simulink model "LAB2_DigitalInput_Output"  (R2024a)
settings: Solver=FixedStepAuto  StartTime=0.0  StopTime=inf  FixedStep=1e-3  RelTol=1e-3  EnableMultiTasking=on
libraries: arduinolib x3
settings Model: ExtModeTrigDuration=2  Creator=VICTUS  LastModifiedBy=VICTUS
settings SolverCC: AutoInsertRateTranBlk=on
settings OptimizationCC: EnhancedBackFolding=on  PassReuseOutputArgsAs=Individual arguments  ZeroExternalMemoryAtStartup=off  ZeroInternalMemoryAtStartup=off  MaxStackSize=64  OptimizeBlockOrder=speed  DifferentSizesBufferReuse=on  OptimizationCustomize=off  EfficientTunableParamExpr=on
settings DebuggingCC: MultiTaskCondExecSysMsg=none  ParameterTunabilityLossMsg=error
settings HardwareCC: ProdBitPerPointer=32  ProdBitPerSizeT=32  ProdBitPerPtrDiffT=32  ProdLargestAtomicInteger=Long  ProdLargestAtomicFloat=Double  ProdWordSize=32  ProdHWDeviceType=ARM Compatible->ARM Cortex
settings SFSimCC: MATLABDynamicMemAlloc=off
settings RTWCC: Description=Embedded Coder  SystemTargetFile=ert.tlc  HardwareBoard=ESP32-WROOM(Arduino Compatible)  TLCOptions="-aInlineSetEventsForThisBaseRateFcn=TLC_FALSE -aSuppressMultiTaskScheduler=TLC_FALSE  -aRateBasedStepFcn=0"  TemplateMakefile=ert_default_tmf  Toolchain=ESP32  BuildConfiguration=Faster Runs
settings CodeAppCC: ForceParamTrailComments=on  IgnoreCustomStorageClasses=off  OperatorAnnotations=on  SimulinkDataObjDesc=on  SFDataObjDesc=on  InsertBlockDesc=on
settings ERTTargetCC: SupportContinuousTime=on  SupportVariableSizeSignals=on  ExtModeTransport=3  ExtModeStaticAlloc=on  ExtModeAutomaticAllocSize=off  ExtModeStaticAllocSize=65536  ExtModeMexFile=ext_xcp  ExtModeIntrfLevel=Level2 - Open

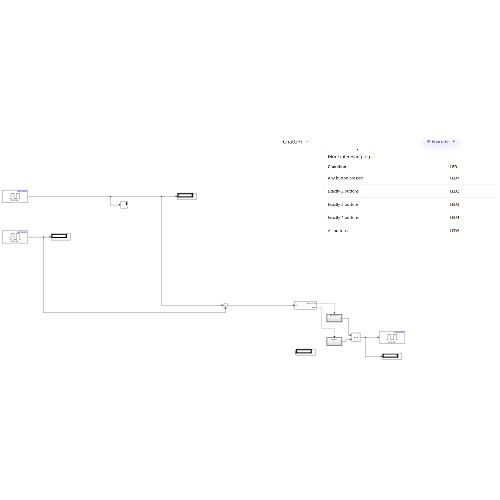
[thumbnail: Simulink's stored preview of the top-level diagram]
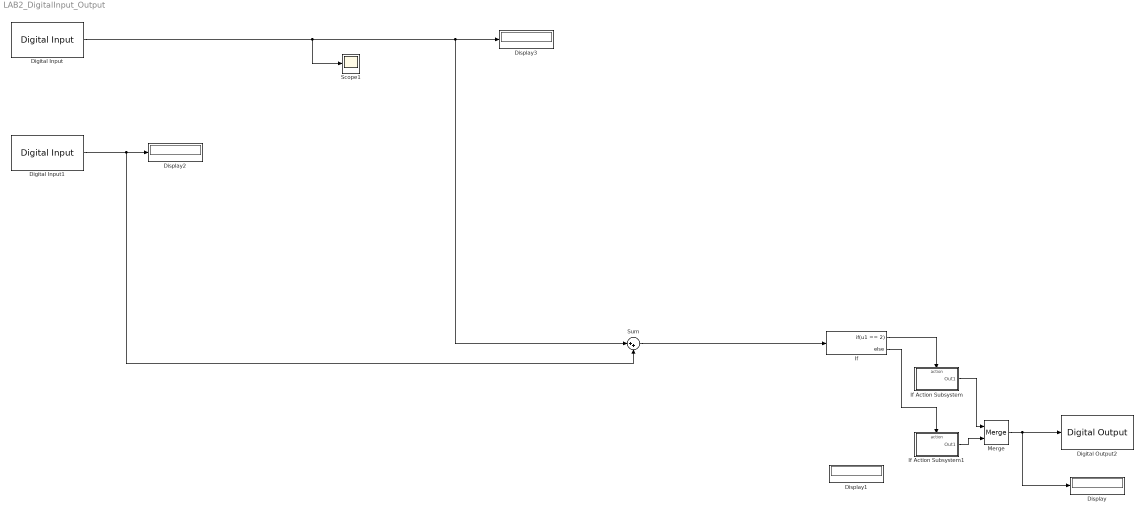
== system LAB2_DigitalInput_Output ==
  Digital Input : arduinolib/Digital Input  pinNumber=25  mode=Default  Direction=input  SampleTime=1E-3  blockPlatform=arduino
  Digital Input1 : arduinolib/Digital Input  pinNumber=34  mode=Default  Direction=input  SampleTime=1E-3  blockPlatform=arduino
  Digital Output2 : arduinolib/Digital Output  pinNumber=23  Direction=output  blockPlatform=arduino
  Display{,1..3} (4 alike) : Display
  If : If  IfExpression=u1 == 2
  If Action Subsystem : Subsystem  TreatAsAtomicUnit=on
  If Action Subsystem1 : Subsystem  TreatAsAtomicUnit=on
  Merge : Merge
  Scope1 : Scope
  Sum : Sum  Inputs=|++
  wires:
  If/1 -> If Action Subsystem/Action
  If Action Subsystem/1(Out1) -> Merge/1
  If/2 -> If Action Subsystem1/Action
  If Action Subsystem1/1(Out1) -> Merge/2
  Merge/1 -> Digital Output2/1, Display/1
  Digital Input/1 -> Sum/1, Display3/1, Scope1/1
  Digital Input1/1 -> Sum/2, Display2/1
  Sum/1 -> If/1

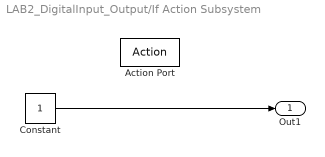
== system LAB2_DigitalInput_Output/If Action Subsystem ==
  Action Port : ActionPort  InitializeStates=reset  ActionPortLabel=if(u1 == 2)
  Constant : Constant
  Out1 : Outport
  wires:
  Constant/1 -> Out1/1

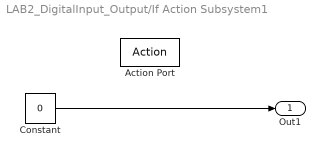
== system LAB2_DigitalInput_Output/If Action Subsystem1 ==
  Action Port : ActionPort  InitializeStates=reset  ActionPortLabel=else
  Constant : Constant  Value=0
  Out1 : Outport
  wires:
  Constant/1 -> Out1/1
